simulink model "SWTTEO"  (R2020a)
settings: Solver=VariableStepAuto  StartTime=0.0  StopTime=20  RelTol=1e-3
libraries: dspsigops x2, dspfdesign x1
settings Model: PauseTimes=2  Creator=diflo  LastModifiedBy=diflo

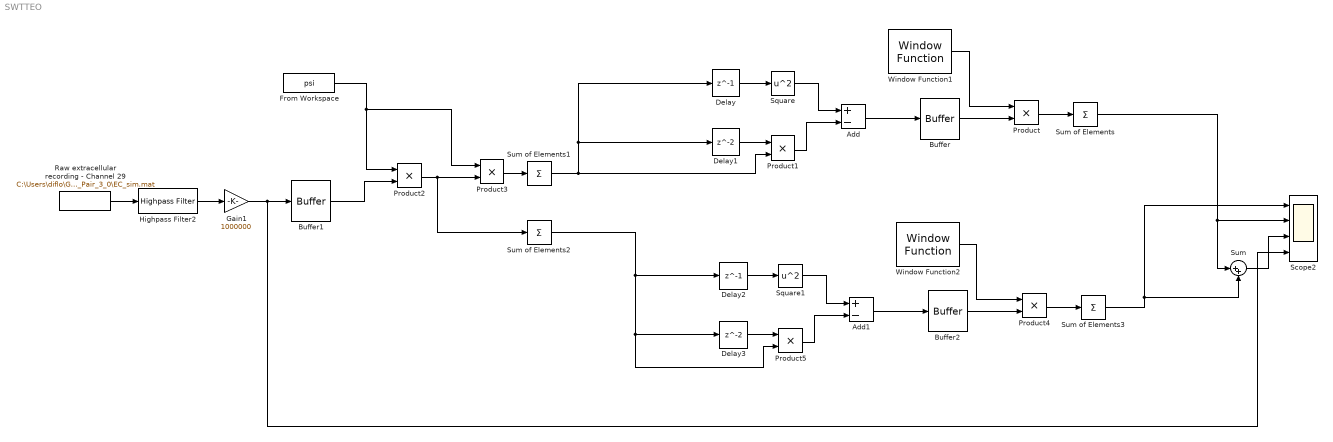
== system SWTTEO ==
  Add : Sum  Inputs=+-
  Add1 : Sum  Inputs=+-
  Buffer : Buffer  N=30  V=29  OutputFrames=off
  Buffer1 : Buffer  N=36  V=35  OutputFrames=off
  Buffer2 : Buffer  N=30  V=29  OutputFrames=off
  Delay : Delay  DelayLength=1  InitialCondition=0  SampleTime=1/30000
  Delay1 : Delay  InitialCondition=0  SampleTime=1/30000
  Delay2 : Delay  DelayLength=1  InitialCondition=0  SampleTime=1/30000
  Delay3 : Delay  InitialCondition=0  SampleTime=1/30000
  From Workspace : FromWorkspace  VariableName=psi  SampleTime=1/30000
  Gain1 : Gain  Gain=1000000
  Highpass Filter2 : dspfdesign/Highpass Filter  FilterType=IIR  DesignForMinimumOrder=off  FilterOrder=3  StopbandFrequency=1  PassbandFrequency=300  StopbandAttenuation=80  PassbandRipple=0.1  InheritSampleRate=off  SampleRate=30000  SimulateUsing=Interpreted execution  roundingMode=Floor  coeffsDataTypeStr=fixdt(1,16)
  Product{,1..5} (6 alike) : Product
  Raw extracellular recording - Channel 29 : FromFile  FileName=C:\Users\diflo\Google Drive\IIT - Neuroengineering\MathWorks Project\Data\KampffLab\2014_11_25_Pair_3_0\EC_sim.mat  SampleTime=1/30000
  Scope2 : Scope  NumInputPorts=4
  Square : Math  Operator=square  SaturateOnIntegerOverflow=on
  Square1 : Math  Operator=square  SaturateOnIntegerOverflow=on
  Sum : Sum  Inputs=|++
  Sum of Elements{,1..3} (4 alike) : Sum  Inputs=+
  Window Function1 : dspsigops/Window Function  winmode=Generate window  wintype=Hamming  sampmode=Discrete  samptime=1/30000  N=30  Rs=50  beta=10  winsamp=Symmetric  UserWindow=hamming  OptParams=off  UserParams={'symmetric'}  dataType=double  isSigned=on  wordLen=16  udDataType=sfix(16)  fracBitsMode=Best precision  numFracBits=15  roundingMode=Floor  overflowMode=off  numSidelobes=4  sidelobeLevel=-30
      settings: SourceProductBaseCode=DS
  Window Function2 : dspsigops/Window Function  winmode=Generate window  wintype=Hamming  sampmode=Discrete  samptime=1/30000  N=30  Rs=50  beta=10  winsamp=Symmetric  UserWindow=hamming  OptParams=off  UserParams={'symmetric'}  dataType=double  isSigned=on  wordLen=16  udDataType=sfix(16)  fracBitsMode=Best precision  numFracBits=15  roundingMode=Floor  overflowMode=off  numSidelobes=4  sidelobeLevel=-30
      settings: SourceProductBaseCode=DS
  wires:
  Raw extracellular recording - Channel 29/1 -> Highpass Filter2/1
  Highpass Filter2/1 -> Gain1/1
  Gain1/1 -> Scope2/4, Buffer1/1
  Buffer1/1 -> Product2/2
  From Workspace/1 -> Product3/1, Product2/1
  Product2/1 -> Product3/2, Sum of Elements2/1
  Product3/1 -> Sum of Elements1/1
  Add/1 -> Buffer/1
  Sum of Elements/1 -> Sum/1, Scope2/2
  Product/1 -> Sum of Elements/1
  Buffer/1 -> Product/2
  Product1/1 -> Add/2
  Delay/1 -> Square/1
  Sum of Elements1/1 -> Product1/2, Delay1/1, Delay/1
  Square/1 -> Add/1
  Window Function1/1 -> Product/1
  Delay1/1 -> Product1/1
  Square1/1 -> Add1/1
  Delay3/1 -> Product5/1
  Window Function2/1 -> Product4/1
  Add1/1 -> Buffer2/1
  Sum of Elements2/1 -> Product5/2, Delay3/1, Delay2/1
  Buffer2/1 -> Product4/2
  Product5/1 -> Add1/2
  Product4/1 -> Sum of Elements3/1
  Delay2/1 -> Square1/1
  Sum of Elements3/1 -> Sum/2, Scope2/1
  Sum/1 -> Scope2/3
